simulink model "receiver_week15"  (R2022a)
settings: Solver=VariableStepAuto  StartTime=0.0  StopTime=inf  RelTol=1e-3
libraries: instrumentseriallib x3
settings Model: Creator=Reaper  LastModifiedBy=Reaper

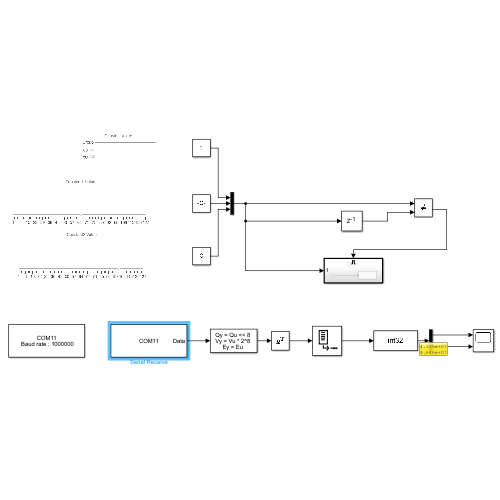
[thumbnail: Simulink's stored preview of the top-level diagram]
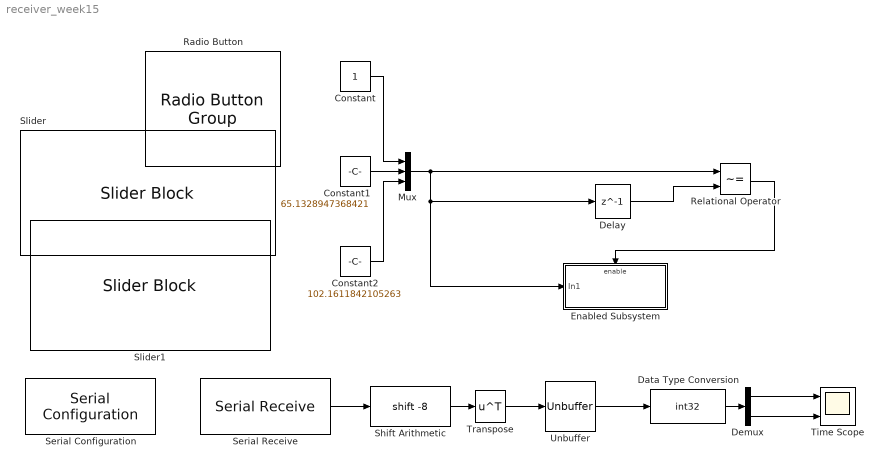
== system receiver_week15 ==
  Constant : Constant  OutDataTypeStr=uint8
  Constant1 : Constant  Value=65.1328947368421  OutDataTypeStr=uint8
  Constant2 : Constant  Value=102.1611842105263  OutDataTypeStr=uint8
  Data Type Conversion : DataTypeConversion  OutDataTypeStr=int32  SaturateOnIntegerOverflow=off  RndMeth=Floor
  Delay : Delay  DelayLength=1
  Demux : Demux  Outputs=2
  Enabled Subsystem : Subsystem  TreatAsAtomicUnit=on
  Mux : Mux  Inputs=3
  Radio Button : RadioButtonGroup  SelectedLabel=ch2  ButtonGroupName=Group
      settings: Values={{'ch1', 'ch2'}, [0 1]}
  Relational Operator : RelationalOperator  Operator=~=  OutDataTypeStr=boolean  RndMeth=Simplest  InputSameDT=off
  Serial Configuration : instrumentseriallib/Serial Configuration  Priority=-200000  PortSel=COM11  Port=COM11  ComPort=COM11  BaudRate=1000000  DataBits=8  Parity=none  StopBits=1  ByteOrder=little-endian  FlowControl=none  Timeout=10  SimulateUsing=Interpreted execution  BlockInModel=on  aMode=1
      settings: SourceProductBaseCode=OT,IC,MT
  Serial Receive : instrumentseriallib/Serial Receive  Priority=1  PortSel=COM11  Port=COM11  ComPort=COM11  DataType=uint32  SaveDataType=uint8  ToggleHeader=on  Header=[83 83]  ToggleTerminator=on  Terminator=Custom terminator  CustomTerminator=[69 69]  InputFormat=Column major  ToggleDataSize=on  DataSize=[2 500]  EnableBlockingMode=on  ActionDataUnavailable=Output last received value  ActionWhenDataUnavailable=Output last received value  CustomValue=0  SampleTime=0.2  SimulateUsing=Interpreted execution  BlockInModel=on  aMode=1
      settings: SourceProductBaseCode=OT,IC,MT
  Shift Arithmetic : ArithShift  BitShiftNumber=-8
  Slider : SliderBlock  ScaleMin=1  ScaleMax=127
  Slider1 : SliderBlock  ScaleMin=1  ScaleMax=127
  Time Scope : Scope  NumInputPorts=2
  Transpose : Math  Operator=transpose
  Unbuffer : Unbuffer
  wires:
  Serial Receive/1 -> Shift Arithmetic/1
  Transpose/1 -> Unbuffer/1
  Unbuffer/1 -> Data Type Conversion/1
  Shift Arithmetic/1 -> Transpose/1
  Data Type Conversion/1 -> Demux/1
  Mux/1 -> Enabled Subsystem/1(In1), Delay/1, Relational Operator/1
  Delay/1 -> Relational Operator/2
  Relational Operator/1 -> Enabled Subsystem/Enable
  Constant2/1 -> Mux/3
  Constant1/1 -> Mux/2
  Constant/1 -> Mux/1
  Demux/1 -> Time Scope/1
  Demux/2 -> Time Scope/2

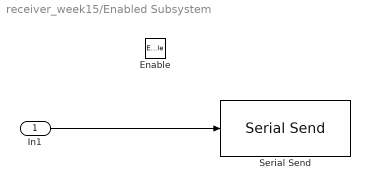
== system receiver_week15/Enabled Subsystem ==
  In1 : Inport
  Enable : EnablePort
  Serial Send : instrumentseriallib/Serial Send  Priority=1  PortSel=COM11  Port=COM11  ComPort=COM11  Header=[]  Terminator=<none>  CustomTerminator=[]  EnableBlockingMode=on  SimulateUsing=Interpreted execution  BlockInModel=on  aMode=1
      settings: SourceProductBaseCode=OT,IC,MT
  wires:
  In1/1 -> Serial Send/1
